simulink model "simulink_example"  (Simulink 7.3)
settings: Solver=ode3  StartTime=0.0  StopTime=10.0  FixedStep=0.004  RelTol=1e-3
values from neighbouring files (symbols this model uses):
  Ac = [0, 1; 0, -1/T]    [create_sys_motor_mat.m]    (also in sys_motor.mat = [0  1; 0  -10])
  Bc = [0; K/T]    [create_sys_motor_mat.m]    (also in sys_motor.mat = [0 2])
libraries: simulink x2
settings Model: Creator=1  LastModifiedBy=1
settings DataIOCC: ReturnWorkspaceOutputs=off
settings DebuggingCC: FcnCallInpInsideContextMsg=Enable All  StrictBusMsg=ErrorLevel1

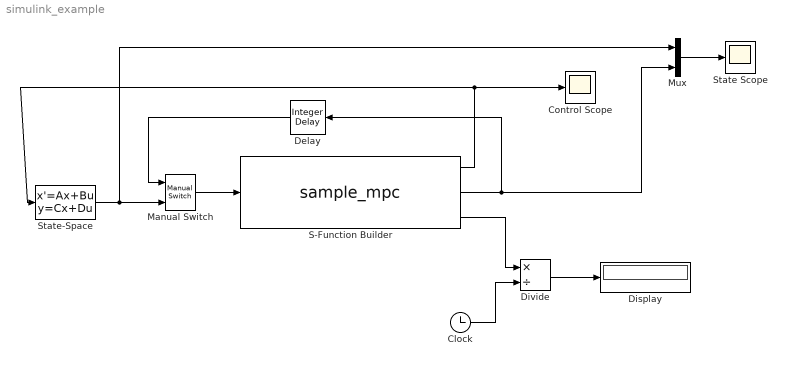
== system simulink_example ==
  Clock : Clock
  Control Scope : Scope
  Delay : simulink/Discrete/Integer Delay  NumDelays=1  vinit=[-1 0]  samptime=-1
  Display : Display
  Divide : Product  Inputs=*/
  Manual Switch : simulink/Signal Routing/Manual Switch  sw=0  action=0  varsize=off
  Mux : Mux  Inputs=2
  S-Function Builder : S-Function  InitFcn=try, set_param(gcb,'FunctionName','sample_mpc'), end  FunctionName=sample_mpc  Parameters=uint32(5)  SFunctionModules=sample_solve_wrapper mtx_ops mpc_const mpc mpc_ref mpc_stc mpc_inc  WizardData=DataTag0  EnableBusSupport=off  mask(S-Function Builder){}
      mask help: Simulink:masks:SFunctionBuilder_MD
      mask init:
      | val = [[.9  0.75 0.75 1 1 .9 .9 1]',[1 1 0.75 0.75 .9 .9 1 .9]'];try , sys = get_param(gcb,'SfunBuilderFcnName');if isempty(sys), sys = get_param(gcb,'FunctionName'); end,catch, sys = get_param(gcb,'FunctionName'); end
      settings: CopyFcn=set_param(gcbh,'LinkStatus','none')  PreSaveFcn=try, set_param(gcb,'FunctionName','sample_mpc'), end  OpenFcn=sfunctionwizard(gcbh)
      mask Display: plot(val(:,1),val(:,2)),disp(sys), port_label('input',1,'x'), port_label('output',1,'u'), port_label('output',2,'x_predicted'), port_label('output',3,'step')
  State Scope : Scope
  State-Space : StateSpace  A=Ac  B=Bc  C=[1 0; 0 1]  D=[0; 0]  X0=[-1; 0]
  wires:
  S-Function Builder/3 -> Divide/1
  Clock/1 -> Divide/2
  Divide/1 -> Display/1
  S-Function Builder/1 -> Control Scope/1, State-Space/1
  State-Space/1 -> Mux/1, Manual Switch/2
  S-Function Builder/2 -> Mux/2, Delay/1
  Manual Switch/1 -> S-Function Builder/1
  Delay/1 -> Manual Switch/1
  Mux/1 -> State Scope/1
